simulink model "sdbe_8_11"  (R2012b)
settings: Solver=VariableStepDiscrete  SolverMode=SingleTasking  StartTime=0.0  StopTime=10000  RelTol=1e-3
PreLoadFcn:
  | counter_vals
undefined symbols (not defined in the file or in its folder): sfp
libraries: xbsIndex_r4 x6687, casper_library_misc x35, casper_library_delays x27, dspsigops x16, xps_library x10, r2dbe_vdif_lib x4, r2dbe_adc_lib x3, simulink x1
(part 21 of 58)

== system sdbe_8_11/quantize_0/scope2 ==
  "data_before " : Inport
  "data_aft " : Inport  Port=2
  Disregard Subsystem : xbsIndex_r4/Disregard Subsystem  Tag=discardX  block_type=disregard
  Gateway Out{,1..7} (8 alike) : xbsIndex_r4/Gateway Out  inherit_from_input=off  hdl_port=on  timing_constraint=None  locs_specified=off  LOCs={}  UseAsDAC=off  DACChannel='1'  block_type=gatewayout
  Mux{,1..3} (4 alike) : Mux  Inputs=2
  Scope{,1..3} (4 alike) : Scope
      Scope settings: YMin=-10  YMax=7.5  SaveName=ScopeData2
      Scope1 settings: YMin=2  YMax=2  SaveName=ScopeData21
      Scope2 settings: YMin=2  YMax=2  SaveName=ScopeData22
      Scope3 settings: YMin=2  YMax=2  SaveName=ScopeData23
  bus_expand : Subsystem  AncestorBlock=casper_library_flow_control/bus_expand  mask(bus_expand){mode=divisions of equal size, outputNum=16, outputWidth=4, outputBinaryPt=0, outputArithmeticType=1, show_format=off, outputToWorkspace=off, variablePrefix=out, outputToModelAsWell=on}
      mask prompts: outputNum "Number of outputs:"; outputWidth "Output width:"; outputBinaryPt "Output binary point position:"; outputArithmeticType "Output arithmetic type (ufix=0, fix=1, bool=2):"; show_format "Print format string?"; outputToWorkspace "Output to workspace?"; variablePrefix "Variable name prefix:"; outputToModelAsWell "Output to model as well?"
      mask help:
      | Expands a 'bus' made using a bus_create or Xilinx
      | concat block.
      | The input will be divided into the specified number
      | of outputs with the specified arithmetic types.
      | Divisions are made from most significant bit.
      mask init: same as sdbe_8_11/get_data_from_pkt/scope/bus_expand1
      settings: AttributesFormatString=16 outputs
      mask TypeOptions mode: divisions of equal size | divisions of arbitrary size
      mask Callback mode: bus_expand_callback();
      mask Callback outputWidth: bus_expand_callback();
      mask Callback outputToWorkspace: bus_expand_callback();
  bus_expand1 : Subsystem  AncestorBlock=casper_library_flow_control/bus_expand  mask(bus_expand){mode=divisions of equal size, outputNum=16, outputWidth=2, outputBinaryPt=0, outputArithmeticType=0, show_format=off, outputToWorkspace=off, variablePrefix=out, outputToModelAsWell=on}
      mask prompts: outputNum "Number of outputs:"; outputWidth "Output width:"; outputBinaryPt "Output binary point position:"; outputArithmeticType "Output arithmetic type (ufix=0, fix=1, bool=2):"; show_format "Print format string?"; outputToWorkspace "Output to workspace?"; variablePrefix "Variable name prefix:"; outputToModelAsWell "Output to model as well?"
      mask help:
      | Expands a 'bus' made using a bus_create or Xilinx
      | concat block.
      | The input will be divided into the specified number
      | of outputs with the specified arithmetic types.
      | Divisions are made from most significant bit.
      mask init: same as sdbe_8_11/get_data_from_pkt/scope/bus_expand1
      settings: AttributesFormatString=16 outputs
      mask TypeOptions mode: divisions of equal size | divisions of arbitrary size
      mask Callback mode: bus_expand_callback();
      mask Callback outputWidth: bus_expand_callback();
      mask Callback outputToWorkspace: bus_expand_callback();
  wires:
  bus_expand/4(out13) -> Gateway Out3/1
  bus_expand/15(out2) -> Gateway Out2/1
  bus_expand/1(msb_out16) -> Gateway Out/1
  Gateway Out2/1 -> [A2]
  bus_expand/16(lsb_out1) -> Gateway Out1/1
  Gateway Out1/1 -> [A3]
  "data_before "/1 -> bus_expand/1(bus_in)
  "data_aft "/1 -> bus_expand1/1(bus_in)
  bus_expand1/1(msb_out16) -> Gateway Out4/1
  Gateway Out4/1 -> Mux/2
  Mux/1 -> Scope/1
  Gateway Out/1 -> [A]
  Gateway Out3/1 -> [A1]
  [A] -> Mux/1
  bus_expand1/4(out13) -> Gateway Out5/1
  Mux1/1 -> Scope1/1
  Gateway Out5/1 -> Mux1/2
  [A1] -> Mux1/1
  bus_expand1/16(lsb_out1) -> Gateway Out6/1
  bus_expand1/15(out2) -> Gateway Out7/1
  Mux2/1 -> Scope2/1
  Gateway Out6/1 -> Mux2/2
  Mux3/1 -> Scope3/1
  Gateway Out7/1 -> Mux3/2
  [A2] -> Mux3/1
  [A3] -> Mux2/1

== system sdbe_8_11/quantize_0/sync_del ==
  d : Inport
  Register0 : xbsIndex_r4/Register  init=0  rst=off  en=off  dbl_ovrd=off  block_type=register
      settings: block_version=11.4
  q : Outport
  wires:
  d/1 -> Register0/1
  Register0/1 -> q/1

== system sdbe_8_11/quantize_0/sync_del1 ==
  d : Inport
  Register0 : xbsIndex_r4/Register  init=0  rst=off  en=off  dbl_ovrd=off  block_type=register
      settings: block_version=11.4
  q : Outport
  wires:
  Register0/1 -> q/1
  d/1 -> Register0/1

== system sdbe_8_11/quantize_0/sync_pipe ==
  d : Inport
  Register0 : xbsIndex_r4/Register  init=0  rst=off  en=off  dbl_ovrd=off  block_type=register
      settings: block_version=11.4
  Register1 : xbsIndex_r4/Register  init=0  rst=off  en=off  dbl_ovrd=off  block_type=register
      settings: block_version=11.4
  Register2 : xbsIndex_r4/Register  init=0  rst=off  en=off  dbl_ovrd=off  block_type=register
      settings: block_version=11.4
  q : Outport
  wires:
  Register2/1 -> q/1
  d/1 -> Register0/1
  Register1/1 -> Register2/1
  Register0/1 -> Register1/1

== system sdbe_8_11/quantize_0/sync_pipe1 ==
  d : Inport
  Register0 : xbsIndex_r4/Register  init=0  rst=off  en=off  dbl_ovrd=off  block_type=register
      settings: block_version=11.4
  Register1 : xbsIndex_r4/Register  init=0  rst=off  en=off  dbl_ovrd=off  block_type=register
      settings: block_version=11.4
  Register2 : xbsIndex_r4/Register  init=0  rst=off  en=off  dbl_ovrd=off  block_type=register
      settings: block_version=11.4
  q : Outport
  wires:
  Register0/1 -> Register1/1
  Register1/1 -> Register2/1
  d/1 -> Register0/1
  Register2/1 -> q/1

== system sdbe_8_11/quantize_0/sync_pipe2 ==
  d : Inport
  Register0 : xbsIndex_r4/Register  init=0  rst=off  en=off  dbl_ovrd=off  block_type=register
      settings: block_version=11.4
  Register1 : xbsIndex_r4/Register  init=0  rst=off  en=off  dbl_ovrd=off  block_type=register
      settings: block_version=11.4
  Register2 : xbsIndex_r4/Register  init=0  rst=off  en=off  dbl_ovrd=off  block_type=register
      settings: block_version=11.4
  q : Outport
  wires:
  Register0/1 -> Register1/1
  Register1/1 -> Register2/1
  d/1 -> Register0/1
  Register2/1 -> q/1

== system sdbe_8_11/quantize_0/sync_pipe3 ==
  d : Inport
  Register0 : xbsIndex_r4/Register  init=0  rst=off  en=off  dbl_ovrd=off  block_type=register
      settings: block_version=11.4
  Register1 : xbsIndex_r4/Register  init=0  rst=off  en=off  dbl_ovrd=off  block_type=register
      settings: block_version=11.4
  Register2 : xbsIndex_r4/Register  init=0  rst=off  en=off  dbl_ovrd=off  block_type=register
      settings: block_version=11.4
  q : Outport
  wires:
  Register2/1 -> q/1
  d/1 -> Register0/1
  Register1/1 -> Register2/1
  Register0/1 -> Register1/1

== system sdbe_8_11/quantize_0/sync_pipe4 ==
  d : Inport
  Register0 : xbsIndex_r4/Register  init=0  rst=off  en=off  dbl_ovrd=off  block_type=register
      settings: block_version=11.4
  Register1 : xbsIndex_r4/Register  init=0  rst=off  en=off  dbl_ovrd=off  block_type=register
      settings: block_version=11.4
  Register2 : xbsIndex_r4/Register  init=0  rst=off  en=off  dbl_ovrd=off  block_type=register
      settings: block_version=11.4
  q : Outport
  wires:
  Register0/1 -> Register1/1
  Register1/1 -> Register2/1
  d/1 -> Register0/1
  Register2/1 -> q/1

== system sdbe_8_11/quantize_0/thr_pipe ==
  d : Inport
  Register0 : xbsIndex_r4/Register  init=0  rst=off  en=off  dbl_ovrd=off  block_type=register
      settings: block_version=11.4
  Register1 : xbsIndex_r4/Register  init=0  rst=off  en=off  dbl_ovrd=off  block_type=register
      settings: block_version=11.4
  Register2 : xbsIndex_r4/Register  init=0  rst=off  en=off  dbl_ovrd=off  block_type=register
      settings: block_version=11.4
  q : Outport
  wires:
  Register2/1 -> q/1
  d/1 -> Register0/1
  Register1/1 -> Register2/1
  Register0/1 -> Register1/1

== system sdbe_8_11/quantize_0/thresh ==
  sim_1 : Inport
  io_delay : xbsIndex_r4/Delay  rst=off  infoeditControl=Selection of Reset will increase slice count due to use of real FFs and instead of SRLs  en=off  latency=0  dbl_ovrd=off  reg_retiming=on  block_type=delay
  reint1 : xbsIndex_r4/Reinterpret  force_arith_type=on  arith_type=Unsigned  force_bin_pt=on  bin_pt=0  block_type=reinterpret
  sdbe_8_11_quantize_0_thresh_user_data_out : xbsIndex_r4/Gateway In  gui_display_data_type=Fixed-point  arith_type=Unsigned  n_bits=32  bin_pt=0  preci_type=Single  exp_width=8  frac_width=24  quantization="Round  (unbiased: +/- Inf)"  overflow=Saturate  period=1  dbl_ovrd=off  timing_constraint=None  locs_specified=off  LOCs={}  UseAsADC=off  ADCChannel='1'  inherit_from_input=off  hdl_port=on  block_type=gatewayin
  slice_gain : xbsIndex_r4/Slice  nbits=32  boolean_output=off  mode=Lower Bit Location + Width  bit1=0  base1=MSB of Input  bit0=0  base0=LSB of Input  dbl_ovrd=off  block_type=slice
  in_gain : Outport
  wires:
  sdbe_8_11_quantize_0_thresh_user_data_out/1 -> io_delay/1
  sim_1/1 -> sdbe_8_11_quantize_0_thresh_user_data_out/1
  io_delay/1 -> slice_gain/1
  slice_gain/1 -> reint1/1
  reint1/1 -> in_gain/1

== system sdbe_8_11/quantize_0/vlbi_2bit ==
  sync_in : Inport
  din : Inport  Port=2
  thresh : Inport  Port=3
  data_val_in : Inport  Port=4
  eof : Inport  Port=5
  hdr : Inport  Port=6
  hdr_valid : Inport  Port=7
  bus_create : Subsystem  AncestorBlock=casper_library_flow_control/bus_create  mask(bus_create){inputNum=16}
      mask prompts: inputNum "Number of inputs:"
      mask init:
      | bus_create_init(gcb,...
      |     'inputNum', inputNum);
  bus_expand : Subsystem  AncestorBlock=casper_library_flow_control/bus_expand  mask(bus_expand){mode=divisions of equal size, outputNum=16, outputWidth=4, outputBinaryPt=0, outputArithmeticType=1, show_format=off, outputToWorkspace=off, variablePrefix=out, outputToModelAsWell=on}
      mask prompts: outputNum "Number of outputs:"; outputWidth "Output width:"; outputBinaryPt "Output binary point position:"; outputArithmeticType "Output arithmetic type (ufix=0, fix=1, bool=2):"; show_format "Print format string?"; outputToWorkspace "Output to workspace?"; variablePrefix "Variable name prefix:"; outputToModelAsWell "Output to model as well?"
      mask help:
      | Expands a 'bus' made using a bus_create or Xilinx
      | concat block.
      | The input will be divided into the specified number
      | of outputs with the specified arithmetic types.
      | Divisions are made from most significant bit.
      mask init: same as sdbe_8_11/get_data_from_pkt/scope/bus_expand1
      settings: AttributesFormatString=16 outputs
      mask TypeOptions mode: divisions of equal size | divisions of arbitrary size
      mask Callback mode: bus_expand_callback();
      mask Callback outputWidth: bus_expand_callback();
      mask Callback outputToWorkspace: bus_expand_callback();
  pipeline : Subsystem  AncestorBlock=casper_library_delays/pipeline  mask(pipeline){latency=3}
      mask help:
      | An explicitly laid-out delay line to avoid mapping to SRL16s
      | for use in pipelining to help achieve timing closure.
      mask init:
      | pipeline_init(gcb,'latency',latency);
      settings: AttributesFormatString=Latency = %<latency>
      mask Display:
      | port_label('input', 1, 'd');
      | port_label('output', 1, 'q');
      | disp(['Z^-', num2str(latency)]);
  pipeline1 : Subsystem  AncestorBlock=casper_library_delays/pipeline  mask(pipeline){latency=3}
      mask help:
      | An explicitly laid-out delay line to avoid mapping to SRL16s
      | for use in pipelining to help achieve timing closure.
      mask init:
      | pipeline_init(gcb,'latency',latency);
      settings: AttributesFormatString=Latency = %<latency>
      mask Display:
      | port_label('input', 1, 'd');
      | port_label('output', 1, 'q');
      | disp(['Z^-', num2str(latency)]);
  pipeline2 : Subsystem  AncestorBlock=casper_library_delays/pipeline  mask(pipeline){latency=3}
      mask help:
      | An explicitly laid-out delay line to avoid mapping to SRL16s
      | for use in pipelining to help achieve timing closure.
      mask init:
      | pipeline_init(gcb,'latency',latency);
      settings: AttributesFormatString=Latency = %<latency>
      mask Display:
      | port_label('input', 1, 'd');
      | port_label('output', 1, 'q');
      | disp(['Z^-', num2str(latency)]);
  pipeline3 : Subsystem  AncestorBlock=casper_library_delays/pipeline  mask(pipeline){latency=3}
      mask help:
      | An explicitly laid-out delay line to avoid mapping to SRL16s
      | for use in pipelining to help achieve timing closure.
      mask init:
      | pipeline_init(gcb,'latency',latency);
      settings: AttributesFormatString=Latency = %<latency>
      mask Display:
      | port_label('input', 1, 'd');
      | port_label('output', 1, 'q');
      | disp(['Z^-', num2str(latency)]);
  pipeline4 : Subsystem  AncestorBlock=casper_library_delays/pipeline  mask(pipeline){latency=3}
      mask help:
      | An explicitly laid-out delay line to avoid mapping to SRL16s
      | for use in pipelining to help achieve timing closure.
      mask init:
      | pipeline_init(gcb,'latency',latency);
      settings: AttributesFormatString=Latency = %<latency>
      mask Display:
      | port_label('input', 1, 'd');
      | port_label('output', 1, 'q');
      | disp(['Z^-', num2str(latency)]);
  quant0 : Subsystem
  quant1 : Subsystem
  quant10 : Subsystem
  quant11 : Subsystem
  quant12 : Subsystem
  quant13 : Subsystem
  quant14 : Subsystem
  quant15 : Subsystem
  quant2 : Subsystem
  quant3 : Subsystem
  quant4 : Subsystem
  quant5 : Subsystem
  quant6 : Subsystem
  quant7 : Subsystem
  quant8 : Subsystem
  quant9 : Subsystem
  sync_out : Outport
  dout : Outport  Port=2
  data_val_out : Outport  Port=3
  eof_out : Outport  Port=4
  hdr_out : Outport  Port=5
  hdr_val_out : Outport  Port=6
  wires:
  pipeline/1(q) -> sync_out/1
  quant10/1(dout2) -> bus_create/11(in11)
  quant15/1(dout2) -> bus_create/16(in16)
  quant8/1(dout2) -> bus_create/9(in9)
  quant11/1(dout2) -> bus_create/12(in12)
  quant12/1(dout2) -> bus_create/13(in13)
  quant9/1(dout2) -> bus_create/10(in10)
  quant14/1(dout2) -> bus_create/15(in15)
  quant13/1(dout2) -> bus_create/14(in14)
  quant5/1(dout2) -> bus_create/6(in6)
  quant4/1(dout2) -> bus_create/5(in5)
  quant7/1(dout2) -> bus_create/8(in8)
  quant6/1(dout2) -> bus_create/7(in7)
  quant2/1(dout2) -> bus_create/3(in3)
  quant3/1(dout2) -> bus_create/4(in4)
  quant1/1(dout2) -> bus_create/2(in2)
  quant0/1(dout2) -> bus_create/1(in1)
  thresh/1 -> quant15/2(thr), quant14/2(thr), quant13/2(thr), quant12/2(thr), quant11/2(thr), quant10/2(thr), quant9/2(thr), quant8/2(thr), quant7/2(thr), quant6/2(thr), quant5/2(thr), quant4/2(thr), quant3/2(thr), quant2/2(thr), quant1/2(thr), quant0/2(thr)
  bus_create/1(bus_out) -> dout/1
  bus_expand/9(out8) -> quant8/1(din4)
  bus_expand/14(out3) -> quant13/1(din4)
  bus_expand/6(out11) -> quant5/1(din4)
  bus_expand/16(lsb_out1) -> quant15/1(din4)
  bus_expand/2(out15) -> quant1/1(din4)
  bus_expand/11(out6) -> quant10/1(din4)
  bus_expand/1(msb_out16) -> quant0/1(din4)
  bus_expand/5(out12) -> quant4/1(din4)
  bus_expand/3(out14) -> quant2/1(din4)
  bus_expand/10(out7) -> quant9/1(din4)
  bus_expand/12(out5) -> quant11/1(din4)
  bus_expand/4(out13) -> quant3/1(din4)
  bus_expand/13(out4) -> quant12/1(din4)
  bus_expand/8(out9) -> quant7/1(din4)
  bus_expand/15(out2) -> quant14/1(din4)
  bus_expand/7(out10) -> quant6/1(din4)
  sync_in/1 -> pipeline/1(d)
  din/1 -> bus_expand/1(bus_in)
  pipeline1/1(q) -> data_val_out/1
  data_val_in/1 -> pipeline1/1(d)
  pipeline2/1(q) -> eof_out/1
  eof/1 -> pipeline2/1(d)
  pipeline3/1(q) -> hdr_out/1
  hdr/1 -> pipeline3/1(d)
  pipeline4/1(q) -> hdr_val_out/1
  hdr_valid/1 -> pipeline4/1(d)

== system sdbe_8_11/quantize_1/din_pipe1 ==
  d : Inport
  Register0 : xbsIndex_r4/Register  init=0  rst=off  en=off  dbl_ovrd=off  block_type=register
      settings: block_version=11.4
  Register1 : xbsIndex_r4/Register  init=0  rst=off  en=off  dbl_ovrd=off  block_type=register
      settings: block_version=11.4
  Register2 : xbsIndex_r4/Register  init=0  rst=off  en=off  dbl_ovrd=off  block_type=register
      settings: block_version=11.4
  q : Outport
  wires:
  Register2/1 -> q/1
  d/1 -> Register0/1
  Register1/1 -> Register2/1
  Register0/1 -> Register1/1

== system sdbe_8_11/quantize_1/eof_del ==
  d : Inport
  Register0 : xbsIndex_r4/Register  init=0  rst=off  en=off  dbl_ovrd=off  block_type=register
      settings: block_version=11.4
  q : Outport
  wires:
  Register0/1 -> q/1
  d/1 -> Register0/1

== system sdbe_8_11/quantize_1/eof_del1 ==
  d : Inport
  Register0 : xbsIndex_r4/Register  init=0  rst=off  en=off  dbl_ovrd=off  block_type=register
      settings: block_version=11.4
  q : Outport
  wires:
  d/1 -> Register0/1
  Register0/1 -> q/1

== system sdbe_8_11/quantize_1/eof_del2 ==
  d : Inport
  Register0 : xbsIndex_r4/Register  init=0  rst=off  en=off  dbl_ovrd=off  block_type=register
      settings: block_version=11.4
  q : Outport
  wires:
  Register0/1 -> q/1
  d/1 -> Register0/1

== system sdbe_8_11/quantize_1/pipeline ==
  d : Inport
  Register0 : xbsIndex_r4/Register  init=0  rst=off  en=off  dbl_ovrd=off  block_type=register
      settings: block_version=11.4
  q : Outport
  wires:
  d/1 -> Register0/1
  Register0/1 -> q/1

== system sdbe_8_11/quantize_1/scope ==
  data : Inport
  valid : Inport  Port=2
  Disregard Subsystem : xbsIndex_r4/Disregard Subsystem  Tag=discardX  block_type=disregard
  Gateway Out{,1..4} (5 alike) : xbsIndex_r4/Gateway Out  inherit_from_input=off  hdl_port=on  timing_constraint=None  locs_specified=off  LOCs={}  UseAsDAC=off  DACChannel='1'  block_type=gatewayout
  Scope{,1..4} (5 alike) : Scope
      Scope settings: YMin=2  YMax=2  SaveName=ScopeData2
      Scope1 settings: SaveName=ScopeData3
      Scope2 settings: SaveName=ScopeData4
      Scope3 settings: SaveName=ScopeData9
      Scope4 settings: SaveName=ScopeData24
  bus_expand : Subsystem  AncestorBlock=casper_library_flow_control/bus_expand  mask(bus_expand){mode=divisions of equal size, outputNum=16, outputWidth=2, outputBinaryPt=0, outputArithmeticType=0, show_format=off, outputToWorkspace=off, variablePrefix=out, outputToModelAsWell=on}
      mask prompts: outputNum "Number of outputs:"; outputWidth "Output width:"; outputBinaryPt "Output binary point position:"; outputArithmeticType "Output arithmetic type (ufix=0, fix=1, bool=2):"; show_format "Print format string?"; outputToWorkspace "Output to workspace?"; variablePrefix "Variable name prefix:"; outputToModelAsWell "Output to model as well?"
      mask help:
      | Expands a 'bus' made using a bus_create or Xilinx
      | concat block.
      | The input will be divided into the specified number
      | of outputs with the specified arithmetic types.
      | Divisions are made from most significant bit.
      mask init: same as sdbe_8_11/get_data_from_pkt/scope/bus_expand1
      settings: AttributesFormatString=16 outputs
      mask TypeOptions mode: divisions of equal size | divisions of arbitrary size
      mask Callback mode: bus_expand_callback();
      mask Callback outputWidth: bus_expand_callback();
      mask Callback outputToWorkspace: bus_expand_callback();
  wires:
  Gateway Out4/1 -> Scope4/1
  valid/1 -> Gateway Out4/1
  bus_expand/4(out13) -> Gateway Out3/1
  Gateway Out3/1 -> Scope3/1
  bus_expand/15(out2) -> Gateway Out2/1
  bus_expand/1(msb_out16) -> Gateway Out/1
  Gateway Out2/1 -> Scope2/1
  bus_expand/16(lsb_out1) -> Gateway Out1/1
  Gateway Out1/1 -> Scope1/1
  Gateway Out/1 -> Scope/1
  data/1 -> bus_expand/1(bus_in)

== system sdbe_8_11/quantize_1/scope1 ==
  data : Inport
  Disregard Subsystem : xbsIndex_r4/Disregard Subsystem  Tag=discardX  block_type=disregard
  Gateway Out{,1..3} (4 alike) : xbsIndex_r4/Gateway Out  inherit_from_input=off  hdl_port=on  timing_constraint=None  locs_specified=off  LOCs={}  UseAsDAC=off  DACChannel='1'  block_type=gatewayout
  Scope{,1..3} (4 alike) : Scope
      Scope settings: YMin=2  YMax=2  SaveName=ScopeData2
      Scope1 settings: SaveName=ScopeData3
      Scope2 settings: SaveName=ScopeData4
      Scope3 settings: SaveName=ScopeData9
  bus_expand : Subsystem  AncestorBlock=casper_library_flow_control/bus_expand  mask(bus_expand){mode=divisions of equal size, outputNum=16, outputWidth=4, outputBinaryPt=0, outputArithmeticType=1, show_format=off, outputToWorkspace=off, variablePrefix=out, outputToModelAsWell=on}
      mask prompts: outputNum "Number of outputs:"; outputWidth "Output width:"; outputBinaryPt "Output binary point position:"; outputArithmeticType "Output arithmetic type (ufix=0, fix=1, bool=2):"; show_format "Print format string?"; outputToWorkspace "Output to workspace?"; variablePrefix "Variable name prefix:"; outputToModelAsWell "Output to model as well?"
      mask help:
      | Expands a 'bus' made using a bus_create or Xilinx
      | concat block.
      | The input will be divided into the specified number
      | of outputs with the specified arithmetic types.
      | Divisions are made from most significant bit.
      mask init: same as sdbe_8_11/get_data_from_pkt/scope/bus_expand1
      settings: AttributesFormatString=16 outputs
      mask TypeOptions mode: divisions of equal size | divisions of arbitrary size
      mask Callback mode: bus_expand_callback();
      mask Callback outputWidth: bus_expand_callback();
      mask Callback outputToWorkspace: bus_expand_callback();
  wires:
  data/1 -> bus_expand/1(bus_in)
  Gateway Out/1 -> Scope/1
  Gateway Out1/1 -> Scope1/1
  bus_expand/16(lsb_out1) -> Gateway Out1/1
  Gateway Out2/1 -> Scope2/1
  bus_expand/1(msb_out16) -> Gateway Out/1
  bus_expand/15(out2) -> Gateway Out2/1
  Gateway Out3/1 -> Scope3/1
  bus_expand/4(out13) -> Gateway Out3/1

== system sdbe_8_11/quantize_1/scope2 ==
  "data_before " : Inport
  "data_aft " : Inport  Port=2
  Disregard Subsystem : xbsIndex_r4/Disregard Subsystem  Tag=discardX  block_type=disregard
  Gateway Out{,1..7} (8 alike) : xbsIndex_r4/Gateway Out  inherit_from_input=off  hdl_port=on  timing_constraint=None  locs_specified=off  LOCs={}  UseAsDAC=off  DACChannel='1'  block_type=gatewayout
  Mux{,1..3} (4 alike) : Mux  Inputs=2
  Scope{,1..3} (4 alike) : Scope
      Scope settings: YMin=-10  YMax=7.5  SaveName=ScopeData2
      Scope1 settings: YMin=2  YMax=2  SaveName=ScopeData21
      Scope2 settings: YMin=2  YMax=2  SaveName=ScopeData22
      Scope3 settings: YMin=2  YMax=2  SaveName=ScopeData23
  bus_expand : Subsystem  AncestorBlock=casper_library_flow_control/bus_expand  mask(bus_expand){mode=divisions of equal size, outputNum=16, outputWidth=4, outputBinaryPt=0, outputArithmeticType=1, show_format=off, outputToWorkspace=off, variablePrefix=out, outputToModelAsWell=on}
      mask prompts: outputNum "Number of outputs:"; outputWidth "Output width:"; outputBinaryPt "Output binary point position:"; outputArithmeticType "Output arithmetic type (ufix=0, fix=1, bool=2):"; show_format "Print format string?"; outputToWorkspace "Output to workspace?"; variablePrefix "Variable name prefix:"; outputToModelAsWell "Output to model as well?"
      mask help:
      | Expands a 'bus' made using a bus_create or Xilinx
      | concat block.
      | The input will be divided into the specified number
      | of outputs with the specified arithmetic types.
      | Divisions are made from most significant bit.
      mask init: same as sdbe_8_11/get_data_from_pkt/scope/bus_expand1
      settings: AttributesFormatString=16 outputs
      mask TypeOptions mode: divisions of equal size | divisions of arbitrary size
      mask Callback mode: bus_expand_callback();
      mask Callback outputWidth: bus_expand_callback();
      mask Callback outputToWorkspace: bus_expand_callback();
  bus_expand1 : Subsystem  AncestorBlock=casper_library_flow_control/bus_expand  mask(bus_expand){mode=divisions of equal size, outputNum=16, outputWidth=2, outputBinaryPt=0, outputArithmeticType=0, show_format=off, outputToWorkspace=off, variablePrefix=out, outputToModelAsWell=on}
      mask prompts: outputNum "Number of outputs:"; outputWidth "Output width:"; outputBinaryPt "Output binary point position:"; outputArithmeticType "Output arithmetic type (ufix=0, fix=1, bool=2):"; show_format "Print format string?"; outputToWorkspace "Output to workspace?"; variablePrefix "Variable name prefix:"; outputToModelAsWell "Output to model as well?"
      mask help:
      | Expands a 'bus' made using a bus_create or Xilinx
      | concat block.
      | The input will be divided into the specified number
      | of outputs with the specified arithmetic types.
      | Divisions are made from most significant bit.
      mask init: same as sdbe_8_11/get_data_from_pkt/scope/bus_expand1
      settings: AttributesFormatString=16 outputs
      mask TypeOptions mode: divisions of equal size | divisions of arbitrary size
      mask Callback mode: bus_expand_callback();
      mask Callback outputWidth: bus_expand_callback();
      mask Callback outputToWorkspace: bus_expand_callback();
  wires:
  [A3] -> Mux2/1
  [A2] -> Mux3/1
  Gateway Out7/1 -> Mux3/2
  Mux3/1 -> Scope3/1
  Gateway Out6/1 -> Mux2/2
  Mux2/1 -> Scope2/1
  bus_expand1/15(out2) -> Gateway Out7/1
  bus_expand1/16(lsb_out1) -> Gateway Out6/1
  [A1] -> Mux1/1
  Gateway Out5/1 -> Mux1/2
  Mux1/1 -> Scope1/1
  bus_expand1/4(out13) -> Gateway Out5/1
  [A] -> Mux/1
  Gateway Out3/1 -> [A1]
  Gateway Out/1 -> [A]
  Mux/1 -> Scope/1
  Gateway Out4/1 -> Mux/2
  bus_expand1/1(msb_out16) -> Gateway Out4/1
  "data_aft "/1 -> bus_expand1/1(bus_in)
  "data_before "/1 -> bus_expand/1(bus_in)
  Gateway Out1/1 -> [A3]
  bus_expand/16(lsb_out1) -> Gateway Out1/1
  Gateway Out2/1 -> [A2]
  bus_expand/1(msb_out16) -> Gateway Out/1
  bus_expand/15(out2) -> Gateway Out2/1
  bus_expand/4(out13) -> Gateway Out3/1

== system sdbe_8_11/quantize_1/sync_del ==
  d : Inport
  Register0 : xbsIndex_r4/Register  init=0  rst=off  en=off  dbl_ovrd=off  block_type=register
      settings: block_version=11.4
  q : Outport
  wires:
  Register0/1 -> q/1
  d/1 -> Register0/1

== system sdbe_8_11/quantize_1/sync_del1 ==
  d : Inport
  Register0 : xbsIndex_r4/Register  init=0  rst=off  en=off  dbl_ovrd=off  block_type=register
      settings: block_version=11.4
  q : Outport
  wires:
  d/1 -> Register0/1
  Register0/1 -> q/1

== system sdbe_8_11/quantize_1/sync_pipe ==
  d : Inport
  Register0 : xbsIndex_r4/Register  init=0  rst=off  en=off  dbl_ovrd=off  block_type=register
      settings: block_version=11.4
  Register1 : xbsIndex_r4/Register  init=0  rst=off  en=off  dbl_ovrd=off  block_type=register
      settings: block_version=11.4
  Register2 : xbsIndex_r4/Register  init=0  rst=off  en=off  dbl_ovrd=off  block_type=register
      settings: block_version=11.4
  q : Outport
  wires:
  Register0/1 -> Register1/1
  Register1/1 -> Register2/1
  d/1 -> Register0/1
  Register2/1 -> q/1

== system sdbe_8_11/quantize_1/sync_pipe1 ==
  d : Inport
  Register0 : xbsIndex_r4/Register  init=0  rst=off  en=off  dbl_ovrd=off  block_type=register
      settings: block_version=11.4
  Register1 : xbsIndex_r4/Register  init=0  rst=off  en=off  dbl_ovrd=off  block_type=register
      settings: block_version=11.4
  Register2 : xbsIndex_r4/Register  init=0  rst=off  en=off  dbl_ovrd=off  block_type=register
      settings: block_version=11.4
  q : Outport
  wires:
  Register2/1 -> q/1
  d/1 -> Register0/1
  Register1/1 -> Register2/1
  Register0/1 -> Register1/1

== system sdbe_8_11/quantize_1/sync_pipe2 ==
  d : Inport
  Register0 : xbsIndex_r4/Register  init=0  rst=off  en=off  dbl_ovrd=off  block_type=register
      settings: block_version=11.4
  Register1 : xbsIndex_r4/Register  init=0  rst=off  en=off  dbl_ovrd=off  block_type=register
      settings: block_version=11.4
  Register2 : xbsIndex_r4/Register  init=0  rst=off  en=off  dbl_ovrd=off  block_type=register
      settings: block_version=11.4
  q : Outport
  wires:
  Register2/1 -> q/1
  d/1 -> Register0/1
  Register1/1 -> Register2/1
  Register0/1 -> Register1/1

== system sdbe_8_11/quantize_1/sync_pipe3 ==
  d : Inport
  Register0 : xbsIndex_r4/Register  init=0  rst=off  en=off  dbl_ovrd=off  block_type=register
      settings: block_version=11.4
  Register1 : xbsIndex_r4/Register  init=0  rst=off  en=off  dbl_ovrd=off  block_type=register
      settings: block_version=11.4
  Register2 : xbsIndex_r4/Register  init=0  rst=off  en=off  dbl_ovrd=off  block_type=register
      settings: block_version=11.4
  q : Outport
  wires:
  Register0/1 -> Register1/1
  Register1/1 -> Register2/1
  d/1 -> Register0/1
  Register2/1 -> q/1

== system sdbe_8_11/quantize_1/sync_pipe4 ==
  d : Inport
  Register0 : xbsIndex_r4/Register  init=0  rst=off  en=off  dbl_ovrd=off  block_type=register
      settings: block_version=11.4
  Register1 : xbsIndex_r4/Register  init=0  rst=off  en=off  dbl_ovrd=off  block_type=register
      settings: block_version=11.4
  Register2 : xbsIndex_r4/Register  init=0  rst=off  en=off  dbl_ovrd=off  block_type=register
      settings: block_version=11.4
  q : Outport
  wires:
  Register2/1 -> q/1
  d/1 -> Register0/1
  Register1/1 -> Register2/1
  Register0/1 -> Register1/1

== system sdbe_8_11/quantize_1/thr_pipe ==
  d : Inport
  Register0 : xbsIndex_r4/Register  init=0  rst=off  en=off  dbl_ovrd=off  block_type=register
      settings: block_version=11.4
  Register1 : xbsIndex_r4/Register  init=0  rst=off  en=off  dbl_ovrd=off  block_type=register
      settings: block_version=11.4
  Register2 : xbsIndex_r4/Register  init=0  rst=off  en=off  dbl_ovrd=off  block_type=register
      settings: block_version=11.4
  q : Outport
  wires:
  Register0/1 -> Register1/1
  Register1/1 -> Register2/1
  d/1 -> Register0/1
  Register2/1 -> q/1

== system sdbe_8_11/quantize_1/thresh ==
  sim_1 : Inport
  io_delay : xbsIndex_r4/Delay  rst=off  infoeditControl=Selection of Reset will increase slice count due to use of real FFs and instead of SRLs  en=off  latency=0  dbl_ovrd=off  reg_retiming=on  block_type=delay
  reint1 : xbsIndex_r4/Reinterpret  force_arith_type=on  arith_type=Unsigned  force_bin_pt=on  bin_pt=0  block_type=reinterpret
  sdbe_8_11_quantize_1_thresh_user_data_out : xbsIndex_r4/Gateway In  gui_display_data_type=Fixed-point  arith_type=Unsigned  n_bits=32  bin_pt=0  preci_type=Single  exp_width=8  frac_width=24  quantization="Round  (unbiased: +/- Inf)"  overflow=Saturate  period=1  dbl_ovrd=off  timing_constraint=None  locs_specified=off  LOCs={}  UseAsADC=off  ADCChannel='1'  inherit_from_input=off  hdl_port=on  block_type=gatewayin
  slice_gain : xbsIndex_r4/Slice  nbits=32  boolean_output=off  mode=Lower Bit Location + Width  bit1=0  base1=MSB of Input  bit0=0  base0=LSB of Input  dbl_ovrd=off  block_type=slice
  in_gain : Outport
  wires:
  sdbe_8_11_quantize_1_thresh_user_data_out/1 -> io_delay/1
  sim_1/1 -> sdbe_8_11_quantize_1_thresh_user_data_out/1
  io_delay/1 -> slice_gain/1
  slice_gain/1 -> reint1/1
  reint1/1 -> in_gain/1

== system sdbe_8_11/quantize_1/vlbi_2bit ==
  sync_in : Inport
  din : Inport  Port=2
  thresh : Inport  Port=3
  data_val_in : Inport  Port=4
  eof : Inport  Port=5
  hdr : Inport  Port=6
  hdr_valid : Inport  Port=7
  bus_create : Subsystem  AncestorBlock=casper_library_flow_control/bus_create  mask(bus_create){inputNum=16}
      mask prompts: inputNum "Number of inputs:"
      mask init:
      | bus_create_init(gcb,...
      |     'inputNum', inputNum);
  bus_expand : Subsystem  AncestorBlock=casper_library_flow_control/bus_expand  mask(bus_expand){mode=divisions of equal size, outputNum=16, outputWidth=4, outputBinaryPt=0, outputArithmeticType=1, show_format=off, outputToWorkspace=off, variablePrefix=out, outputToModelAsWell=on}
      mask prompts: outputNum "Number of outputs:"; outputWidth "Output width:"; outputBinaryPt "Output binary point position:"; outputArithmeticType "Output arithmetic type (ufix=0, fix=1, bool=2):"; show_format "Print format string?"; outputToWorkspace "Output to workspace?"; variablePrefix "Variable name prefix:"; outputToModelAsWell "Output to model as well?"
      mask help:
      | Expands a 'bus' made using a bus_create or Xilinx
      | concat block.
      | The input will be divided into the specified number
      | of outputs with the specified arithmetic types.
      | Divisions are made from most significant bit.
      mask init: same as sdbe_8_11/get_data_from_pkt/scope/bus_expand1
      settings: AttributesFormatString=16 outputs
      mask TypeOptions mode: divisions of equal size | divisions of arbitrary size
      mask Callback mode: bus_expand_callback();
      mask Callback outputWidth: bus_expand_callback();
      mask Callback outputToWorkspace: bus_expand_callback();
  pipeline : Subsystem  AncestorBlock=casper_library_delays/pipeline  mask(pipeline){latency=3}
      mask help:
      | An explicitly laid-out delay line to avoid mapping to SRL16s
      | for use in pipelining to help achieve timing closure.
      mask init:
      | pipeline_init(gcb,'latency',latency);
      settings: AttributesFormatString=Latency = %<latency>
      mask Display:
      | port_label('input', 1, 'd');
      | port_label('output', 1, 'q');
      | disp(['Z^-', num2str(latency)]);
  pipeline1 : Subsystem  AncestorBlock=casper_library_delays/pipeline  mask(pipeline){latency=3}
      mask help:
      | An explicitly laid-out delay line to avoid mapping to SRL16s
      | for use in pipelining to help achieve timing closure.
      mask init:
      | pipeline_init(gcb,'latency',latency);
      settings: AttributesFormatString=Latency = %<latency>
      mask Display:
      | port_label('input', 1, 'd');
      | port_label('output', 1, 'q');
      | disp(['Z^-', num2str(latency)]);
  pipeline2 : Subsystem  AncestorBlock=casper_library_delays/pipeline  mask(pipeline){latency=3}
      mask help:
      | An explicitly laid-out delay line to avoid mapping to SRL16s
      | for use in pipelining to help achieve timing closure.
      mask init:
      | pipeline_init(gcb,'latency',latency);
      settings: AttributesFormatString=Latency = %<latency>
      mask Display:
      | port_label('input', 1, 'd');
      | port_label('output', 1, 'q');
      | disp(['Z^-', num2str(latency)]);
  pipeline3 : Subsystem  AncestorBlock=casper_library_delays/pipeline  mask(pipeline){latency=3}
      mask help:
      | An explicitly laid-out delay line to avoid mapping to SRL16s
      | for use in pipelining to help achieve timing closure.
      mask init:
      | pipeline_init(gcb,'latency',latency);
      settings: AttributesFormatString=Latency = %<latency>
      mask Display:
      | port_label('input', 1, 'd');
      | port_label('output', 1, 'q');
      | disp(['Z^-', num2str(latency)]);
  pipeline4 : Subsystem  AncestorBlock=casper_library_delays/pipeline  mask(pipeline){latency=3}
      mask help:
      | An explicitly laid-out delay line to avoid mapping to SRL16s
      | for use in pipelining to help achieve timing closure.
      mask init:
      | pipeline_init(gcb,'latency',latency);
      settings: AttributesFormatString=Latency = %<latency>
      mask Display:
      | port_label('input', 1, 'd');
      | port_label('output', 1, 'q');
      | disp(['Z^-', num2str(latency)]);
  quant0 : Subsystem
  quant1 : Subsystem
  quant10 : Subsystem
  quant11 : Subsystem
  quant12 : Subsystem
  quant13 : Subsystem
  quant14 : Subsystem
  quant15 : Subsystem
  quant2 : Subsystem
  quant3 : Subsystem
  quant4 : Subsystem
  quant5 : Subsystem
  quant6 : Subsystem
  quant7 : Subsystem
  quant8 : Subsystem
  quant9 : Subsystem
  sync_out : Outport
  dout : Outport  Port=2
  data_val_out : Outport  Port=3
  eof_out : Outport  Port=4
  hdr_out : Outport  Port=5
  hdr_val_out : Outport  Port=6
  wires:
  hdr_valid/1 -> pipeline4/1(d)
  pipeline4/1(q) -> hdr_val_out/1
  hdr/1 -> pipeline3/1(d)
  pipeline3/1(q) -> hdr_out/1
  eof/1 -> pipeline2/1(d)
  pipeline2/1(q) -> eof_out/1
  data_val_in/1 -> pipeline1/1(d)
  pipeline1/1(q) -> data_val_out/1
  din/1 -> bus_expand/1(bus_in)
  sync_in/1 -> pipeline/1(d)
  bus_expand/7(out10) -> quant6/1(din4)
  bus_expand/15(out2) -> quant14/1(din4)
  bus_expand/8(out9) -> quant7/1(din4)
  bus_expand/13(out4) -> quant12/1(din4)
  bus_expand/4(out13) -> quant3/1(din4)
  bus_expand/12(out5) -> quant11/1(din4)
  bus_expand/10(out7) -> quant9/1(din4)
  bus_expand/3(out14) -> quant2/1(din4)
  bus_expand/5(out12) -> quant4/1(din4)
  bus_expand/1(msb_out16) -> quant0/1(din4)
  bus_expand/11(out6) -> quant10/1(din4)
  bus_expand/2(out15) -> quant1/1(din4)
  bus_expand/16(lsb_out1) -> quant15/1(din4)
  bus_expand/6(out11) -> quant5/1(din4)
  bus_expand/14(out3) -> quant13/1(din4)
  bus_expand/9(out8) -> quant8/1(din4)
  bus_create/1(bus_out) -> dout/1
  thresh/1 -> quant0/2(thr), quant1/2(thr), quant2/2(thr), quant3/2(thr), quant4/2(thr), quant5/2(thr), quant6/2(thr), quant7/2(thr), quant8/2(thr), quant9/2(thr), quant10/2(thr), quant11/2(thr), quant12/2(thr), quant13/2(thr), quant14/2(thr), quant15/2(thr)
  quant0/1(dout2) -> bus_create/1(in1)
  quant1/1(dout2) -> bus_create/2(in2)
  quant3/1(dout2) -> bus_create/4(in4)
  quant2/1(dout2) -> bus_create/3(in3)
  quant6/1(dout2) -> bus_create/7(in7)
  quant7/1(dout2) -> bus_create/8(in8)
  quant4/1(dout2) -> bus_create/5(in5)
  quant5/1(dout2) -> bus_create/6(in6)
  quant13/1(dout2) -> bus_create/14(in14)
  quant14/1(dout2) -> bus_create/15(in15)
  quant9/1(dout2) -> bus_create/10(in10)
  quant12/1(dout2) -> bus_create/13(in13)
  quant11/1(dout2) -> bus_create/12(in12)
  quant8/1(dout2) -> bus_create/9(in9)
  quant15/1(dout2) -> bus_create/16(in16)
  quant10/1(dout2) -> bus_create/11(in11)
  pipeline/1(q) -> sync_out/1

== system sdbe_8_11/quantize_2/din_pipe1 ==
  d : Inport
  Register0 : xbsIndex_r4/Register  init=0  rst=off  en=off  dbl_ovrd=off  block_type=register
      settings: block_version=11.4
  Register1 : xbsIndex_r4/Register  init=0  rst=off  en=off  dbl_ovrd=off  block_type=register
      settings: block_version=11.4
  Register2 : xbsIndex_r4/Register  init=0  rst=off  en=off  dbl_ovrd=off  block_type=register
      settings: block_version=11.4
  q : Outport
  wires:
  Register0/1 -> Register1/1
  Register1/1 -> Register2/1
  d/1 -> Register0/1
  Register2/1 -> q/1

== system sdbe_8_11/quantize_2/eof_del ==
  d : Inport
  Register0 : xbsIndex_r4/Register  init=0  rst=off  en=off  dbl_ovrd=off  block_type=register
      settings: block_version=11.4
  q : Outport
  wires:
  d/1 -> Register0/1
  Register0/1 -> q/1

== system sdbe_8_11/quantize_2/eof_del1 ==
  d : Inport
  Register0 : xbsIndex_r4/Register  init=0  rst=off  en=off  dbl_ovrd=off  block_type=register
      settings: block_version=11.4
  q : Outport
  wires:
  Register0/1 -> q/1
  d/1 -> Register0/1

== system sdbe_8_11/quantize_2/eof_del2 ==
  d : Inport
  Register0 : xbsIndex_r4/Register  init=0  rst=off  en=off  dbl_ovrd=off  block_type=register
      settings: block_version=11.4
  q : Outport
  wires:
  d/1 -> Register0/1
  Register0/1 -> q/1

== system sdbe_8_11/quantize_2/pipeline ==
  d : Inport
  Register0 : xbsIndex_r4/Register  init=0  rst=off  en=off  dbl_ovrd=off  block_type=register
      settings: block_version=11.4
  q : Outport
  wires:
  Register0/1 -> q/1
  d/1 -> Register0/1

== system sdbe_8_11/quantize_2/scope ==
  data : Inport
  valid : Inport  Port=2
  Disregard Subsystem : xbsIndex_r4/Disregard Subsystem  Tag=discardX  block_type=disregard
  Gateway Out{,1..4} (5 alike) : xbsIndex_r4/Gateway Out  inherit_from_input=off  hdl_port=on  timing_constraint=None  locs_specified=off  LOCs={}  UseAsDAC=off  DACChannel='1'  block_type=gatewayout
  Scope{,1..4} (5 alike) : Scope
      Scope settings: YMin=2  YMax=2  SaveName=ScopeData2
      Scope1 settings: SaveName=ScopeData3
      Scope2 settings: SaveName=ScopeData4
      Scope3 settings: SaveName=ScopeData9
      Scope4 settings: SaveName=ScopeData24
  bus_expand : Subsystem  AncestorBlock=casper_library_flow_control/bus_expand  mask(bus_expand){mode=divisions of equal size, outputNum=16, outputWidth=2, outputBinaryPt=0, outputArithmeticType=0, show_format=off, outputToWorkspace=off, variablePrefix=out, outputToModelAsWell=on}
      mask prompts: outputNum "Number of outputs:"; outputWidth "Output width:"; outputBinaryPt "Output binary point position:"; outputArithmeticType "Output arithmetic type (ufix=0, fix=1, bool=2):"; show_format "Print format string?"; outputToWorkspace "Output to workspace?"; variablePrefix "Variable name prefix:"; outputToModelAsWell "Output to model as well?"
      mask help:
      | Expands a 'bus' made using a bus_create or Xilinx
      | concat block.
      | The input will be divided into the specified number
      | of outputs with the specified arithmetic types.
      | Divisions are made from most significant bit.
      mask init: same as sdbe_8_11/get_data_from_pkt/scope/bus_expand1
      settings: AttributesFormatString=16 outputs
      mask TypeOptions mode: divisions of equal size | divisions of arbitrary size
      mask Callback mode: bus_expand_callback();
      mask Callback outputWidth: bus_expand_callback();
      mask Callback outputToWorkspace: bus_expand_callback();
  wires:
  data/1 -> bus_expand/1(bus_in)
  Gateway Out/1 -> Scope/1
  Gateway Out1/1 -> Scope1/1
  bus_expand/16(lsb_out1) -> Gateway Out1/1
  Gateway Out2/1 -> Scope2/1
  bus_expand/1(msb_out16) -> Gateway Out/1
  bus_expand/15(out2) -> Gateway Out2/1
  Gateway Out3/1 -> Scope3/1
  bus_expand/4(out13) -> Gateway Out3/1
  valid/1 -> Gateway Out4/1
  Gateway Out4/1 -> Scope4/1

== system sdbe_8_11/quantize_2/scope1 ==
  data : Inport
  Disregard Subsystem : xbsIndex_r4/Disregard Subsystem  Tag=discardX  block_type=disregard
  Gateway Out{,1..3} (4 alike) : xbsIndex_r4/Gateway Out  inherit_from_input=off  hdl_port=on  timing_constraint=None  locs_specified=off  LOCs={}  UseAsDAC=off  DACChannel='1'  block_type=gatewayout
  Scope{,1..3} (4 alike) : Scope
      Scope settings: YMin=2  YMax=2  SaveName=ScopeData2
      Scope1 settings: SaveName=ScopeData3
      Scope2 settings: SaveName=ScopeData4
      Scope3 settings: SaveName=ScopeData9
  bus_expand : Subsystem  AncestorBlock=casper_library_flow_control/bus_expand  mask(bus_expand){mode=divisions of equal size, outputNum=16, outputWidth=4, outputBinaryPt=0, outputArithmeticType=1, show_format=off, outputToWorkspace=off, variablePrefix=out, outputToModelAsWell=on}
      mask prompts: outputNum "Number of outputs:"; outputWidth "Output width:"; outputBinaryPt "Output binary point position:"; outputArithmeticType "Output arithmetic type (ufix=0, fix=1, bool=2):"; show_format "Print format string?"; outputToWorkspace "Output to workspace?"; variablePrefix "Variable name prefix:"; outputToModelAsWell "Output to model as well?"
      mask help:
      | Expands a 'bus' made using a bus_create or Xilinx
      | concat block.
      | The input will be divided into the specified number
      | of outputs with the specified arithmetic types.
      | Divisions are made from most significant bit.
      mask init: same as sdbe_8_11/get_data_from_pkt/scope/bus_expand1
      settings: AttributesFormatString=16 outputs
      mask TypeOptions mode: divisions of equal size | divisions of arbitrary size
      mask Callback mode: bus_expand_callback();
      mask Callback outputWidth: bus_expand_callback();
      mask Callback outputToWorkspace: bus_expand_callback();
  wires:
  bus_expand/4(out13) -> Gateway Out3/1
  Gateway Out3/1 -> Scope3/1
  bus_expand/15(out2) -> Gateway Out2/1
  bus_expand/1(msb_out16) -> Gateway Out/1
  Gateway Out2/1 -> Scope2/1
  bus_expand/16(lsb_out1) -> Gateway Out1/1
  Gateway Out1/1 -> Scope1/1
  Gateway Out/1 -> Scope/1
  data/1 -> bus_expand/1(bus_in)

== system sdbe_8_11/quantize_2/scope2 ==
  "data_before " : Inport
  "data_aft " : Inport  Port=2
  Disregard Subsystem : xbsIndex_r4/Disregard Subsystem  Tag=discardX  block_type=disregard
  Gateway Out{,1..7} (8 alike) : xbsIndex_r4/Gateway Out  inherit_from_input=off  hdl_port=on  timing_constraint=None  locs_specified=off  LOCs={}  UseAsDAC=off  DACChannel='1'  block_type=gatewayout
  Mux{,1..3} (4 alike) : Mux  Inputs=2
  Scope{,1..3} (4 alike) : Scope
      Scope settings: YMin=-10  YMax=7.5  SaveName=ScopeData2
      Scope1 settings: YMin=2  YMax=2  SaveName=ScopeData21
      Scope2 settings: YMin=2  YMax=2  SaveName=ScopeData22
      Scope3 settings: YMin=2  YMax=2  SaveName=ScopeData23
  bus_expand : Subsystem  AncestorBlock=casper_library_flow_control/bus_expand  mask(bus_expand){mode=divisions of equal size, outputNum=16, outputWidth=4, outputBinaryPt=0, outputArithmeticType=1, show_format=off, outputToWorkspace=off, variablePrefix=out, outputToModelAsWell=on}
      mask prompts: outputNum "Number of outputs:"; outputWidth "Output width:"; outputBinaryPt "Output binary point position:"; outputArithmeticType "Output arithmetic type (ufix=0, fix=1, bool=2):"; show_format "Print format string?"; outputToWorkspace "Output to workspace?"; variablePrefix "Variable name prefix:"; outputToModelAsWell "Output to model as well?"
      mask help:
      | Expands a 'bus' made using a bus_create or Xilinx
      | concat block.
      | The input will be divided into the specified number
      | of outputs with the specified arithmetic types.
      | Divisions are made from most significant bit.
      mask init: same as sdbe_8_11/get_data_from_pkt/scope/bus_expand1
      settings: AttributesFormatString=16 outputs
      mask TypeOptions mode: divisions of equal size | divisions of arbitrary size
      mask Callback mode: bus_expand_callback();
      mask Callback outputWidth: bus_expand_callback();
      mask Callback outputToWorkspace: bus_expand_callback();
  bus_expand1 : Subsystem  AncestorBlock=casper_library_flow_control/bus_expand  mask(bus_expand){mode=divisions of equal size, outputNum=16, outputWidth=2, outputBinaryPt=0, outputArithmeticType=0, show_format=off, outputToWorkspace=off, variablePrefix=out, outputToModelAsWell=on}
      mask prompts: outputNum "Number of outputs:"; outputWidth "Output width:"; outputBinaryPt "Output binary point position:"; outputArithmeticType "Output arithmetic type (ufix=0, fix=1, bool=2):"; show_format "Print format string?"; outputToWorkspace "Output to workspace?"; variablePrefix "Variable name prefix:"; outputToModelAsWell "Output to model as well?"
      mask help:
      | Expands a 'bus' made using a bus_create or Xilinx
      | concat block.
      | The input will be divided into the specified number
      | of outputs with the specified arithmetic types.
      | Divisions are made from most significant bit.
      mask init: same as sdbe_8_11/get_data_from_pkt/scope/bus_expand1
      settings: AttributesFormatString=16 outputs
      mask TypeOptions mode: divisions of equal size | divisions of arbitrary size
      mask Callback mode: bus_expand_callback();
      mask Callback outputWidth: bus_expand_callback();
      mask Callback outputToWorkspace: bus_expand_callback();
  wires:
  bus_expand/4(out13) -> Gateway Out3/1
  bus_expand/15(out2) -> Gateway Out2/1
  bus_expand/1(msb_out16) -> Gateway Out/1
  Gateway Out2/1 -> [A2]
  bus_expand/16(lsb_out1) -> Gateway Out1/1
  Gateway Out1/1 -> [A3]
  "data_before "/1 -> bus_expand/1(bus_in)
  "data_aft "/1 -> bus_expand1/1(bus_in)
  bus_expand1/1(msb_out16) -> Gateway Out4/1
  Gateway Out4/1 -> Mux/2
  Mux/1 -> Scope/1
  Gateway Out/1 -> [A]
  Gateway Out3/1 -> [A1]
  [A] -> Mux/1
  bus_expand1/4(out13) -> Gateway Out5/1
  Mux1/1 -> Scope1/1
  Gateway Out5/1 -> Mux1/2
  [A1] -> Mux1/1
  bus_expand1/16(lsb_out1) -> Gateway Out6/1
  bus_expand1/15(out2) -> Gateway Out7/1
  Mux2/1 -> Scope2/1
  Gateway Out6/1 -> Mux2/2
  Mux3/1 -> Scope3/1
  Gateway Out7/1 -> Mux3/2
  [A2] -> Mux3/1
  [A3] -> Mux2/1

== system sdbe_8_11/quantize_2/sync_del ==
  d : Inport
  Register0 : xbsIndex_r4/Register  init=0  rst=off  en=off  dbl_ovrd=off  block_type=register
      settings: block_version=11.4
  q : Outport
  wires:
  d/1 -> Register0/1
  Register0/1 -> q/1

== system sdbe_8_11/quantize_2/sync_del1 ==
  d : Inport
  Register0 : xbsIndex_r4/Register  init=0  rst=off  en=off  dbl_ovrd=off  block_type=register
      settings: block_version=11.4
  q : Outport
  wires:
  Register0/1 -> q/1
  d/1 -> Register0/1

== system sdbe_8_11/quantize_2/sync_pipe ==
  d : Inport
  Register0 : xbsIndex_r4/Register  init=0  rst=off  en=off  dbl_ovrd=off  block_type=register
      settings: block_version=11.4
  Register1 : xbsIndex_r4/Register  init=0  rst=off  en=off  dbl_ovrd=off  block_type=register
      settings: block_version=11.4
  Register2 : xbsIndex_r4/Register  init=0  rst=off  en=off  dbl_ovrd=off  block_type=register
      settings: block_version=11.4
  q : Outport
  wires:
  Register2/1 -> q/1
  d/1 -> Register0/1
  Register1/1 -> Register2/1
  Register0/1 -> Register1/1

== system sdbe_8_11/quantize_2/sync_pipe1 ==
  d : Inport
  Register0 : xbsIndex_r4/Register  init=0  rst=off  en=off  dbl_ovrd=off  block_type=register
      settings: block_version=11.4
  Register1 : xbsIndex_r4/Register  init=0  rst=off  en=off  dbl_ovrd=off  block_type=register
      settings: block_version=11.4
  Register2 : xbsIndex_r4/Register  init=0  rst=off  en=off  dbl_ovrd=off  block_type=register
      settings: block_version=11.4
  q : Outport
  wires:
  Register0/1 -> Register1/1
  Register1/1 -> Register2/1
  d/1 -> Register0/1
  Register2/1 -> q/1
